simulink model "Problem_Simulation"  (R2023b)
settings: Solver=VariableStepAuto  StartTime=0.0  StopTime=1  RelTol=1e-3
libraries: spsDiodeLib x4, spsSeriesRLCBranchLib x2, spsTHDLib x2, spsVoltageMeasurementLib x2, spsACVoltageSourceLib x1, spsCurrentMeasurementLib x1, spsMeanLib x1, spsPowerLib x1, sps_lib x1
settings Model: Creator=HP  LastModifiedBy=HP

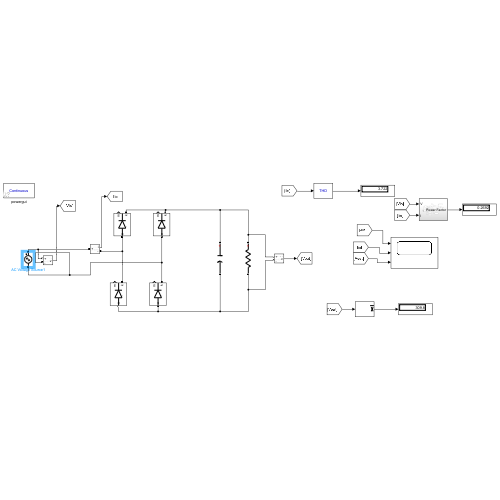
[thumbnail: Simulink's stored preview of the top-level diagram]
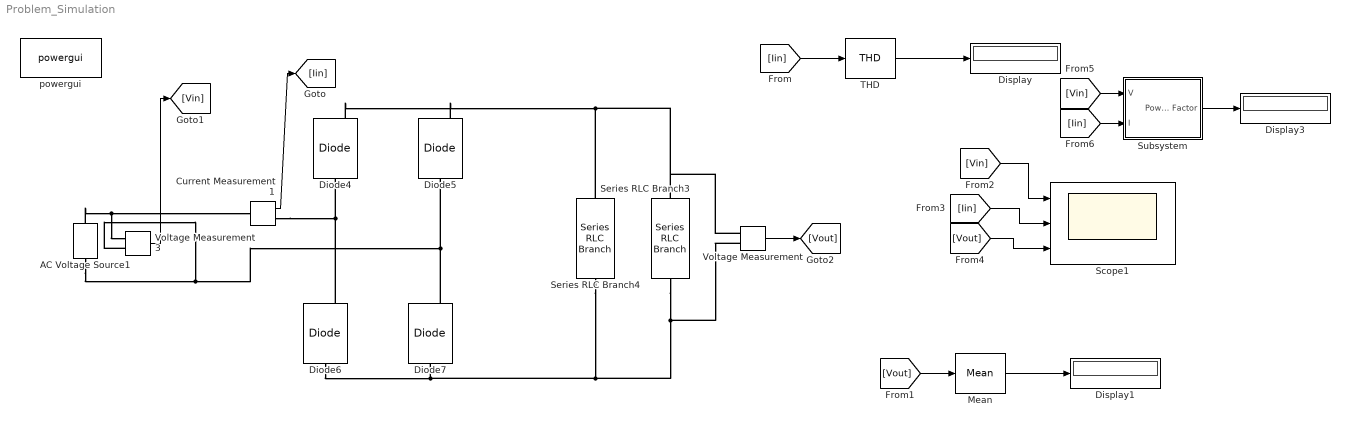
== system Problem_Simulation ==
  AC Voltage Source1 : spsACVoltageSourceLib/AC Voltage Source  Amplitude=220*sqrt(2)  Phase=0  Frequency=50  SampleTime=0  Measurements=None  BusType=swing  Pref=10e3  Qref=0  Qmin=-inf  Qmax=+inf
  Current Measurement1 : spsCurrentMeasurementLib/Current Measurement  PhasorSimulation=off  OutputType=Complex  PSBequivalent=0
  Diode{4..7} (4 alike) : spsDiodeLib/Diode  Ron=0.001  Lon=0  Vf=0.8  IC=0  UseSnubber=0  Rs=500  Cs=250e-9  Measurements=on
  Display : Display
  Display1 : Display
  Display3 : Display
  Mean : spsMeanLib/Mean  Freq=60  Vinit=0  Ts=0
  Scope1 : Scope  NumInputPorts=3
  Series RLC Branch3 : spsSeriesRLCBranchLib/Series RLC Branch  LConnTagsString=__new0  RConnTagsString=__new0  BranchType=R  Resistance=1000  Inductance=1e-3  SetiL0=off  InitialCurrent=0  Capacitance=1e-6  Setx0=off  InitialVoltage=0  Measurements=None
  Series RLC Branch4 : spsSeriesRLCBranchLib/Series RLC Branch  LConnTagsString=__new0  RConnTagsString=__new0  BranchType=C  Resistance=1  Inductance=1e-3  SetiL0=off  InitialCurrent=0  Capacitance=1000e-6  Setx0=off  InitialVoltage=0  Measurements=None
  Subsystem : Subsystem
  THD : spsTHDLib/THD  Freq=50  Ts=0
  Voltage Measurement : spsVoltageMeasurementLib/Voltage Measurement  PhasorSimulation=off  OutputType=Complex  PSBequivalent=0
  Voltage Measurement3 : spsVoltageMeasurementLib/Voltage Measurement  PhasorSimulation=off  OutputType=Complex  PSBequivalent=0
  powergui : sps_lib/powergui  Priority=1  SimulationMode=Continuous  SampleTime=50e-6  frequency=60  Iterations=50  frequencyindice=50  Pbase=100e6  ErrMax=1e-4  UnitsV=kV  UnitsW=MW  buscounter=0  FunctionMessages=off  echomessages=off  EnableUseOfTLC=off  CurrentSourceSwitches=off  DisableSnubberDevices=on  DisableRonSwitches=off  DisableVfSwitches=on  DisplayEquations=on  AutomaticDiscreteSolvers=off  SolverType=Tustin/Backward Euler (TBE)  Interpol=off  ExternalGateDelay=off  methode=off  Ts=100  x0status=blocks  SPID=on  SwTol=0  HookPort=off  NonlinearTolerance=1e-4  nMaxIteration=100  ContinueOnMaxIteration=off  RestoreLinks=warning  ResistiveCurrentMeasurement=off  Frange=[0:2:500]  Ylog=off  Xlog=on  ShowGrid=off  save=off  variable=ZData  structure=0  ZoomFFT=off  StartTime=0.0  cycles=1  DisplayStyle=1  fundamental=60  FreqAxis=off  MaxFrequency=1000  frequencyindicesteady=1  RmsSteady=1  display=off
  wires:
  THD/1 -> Display/1
  Subsystem/1(Power Factor) -> Display3/1
  Mean/1 -> Display1/1
  Current Measurement1/1 -> [Iin]
  [Iin] -> THD/1
  Voltage Measurement3/1 -> [Vin]
  Voltage Measurement/1 -> [Vout]
  [Vout] -> Mean/1
  [Vin] -> Scope1/1
  [Iin] -> Scope1/2
  [Vout] -> Scope1/3
  [Vin] -> Subsystem/1(V)
  [Iin] -> Subsystem/2(I)
  connections:
  Current Measurement1/RConn1 -- Diode4/LConn1 -- Diode6/RConn1
  Diode5/RConn1 -- Diode4/RConn1 -- Voltage Measurement/LConn1 -- Series RLC Branch3/LConn1 -- Series RLC Branch4/LConn1
  Series RLC Branch3/RConn1 -- Voltage Measurement/LConn2 -- Series RLC Branch4/RConn1 -- Diode7/LConn1 -- Diode6/LConn1
  AC Voltage Source1/RConn1 -- Voltage Measurement3/LConn1 -- Current Measurement1/LConn1
  AC Voltage Source1/LConn1 -- Voltage Measurement3/LConn2 -- Diode5/LConn1 -- Diode7/RConn1

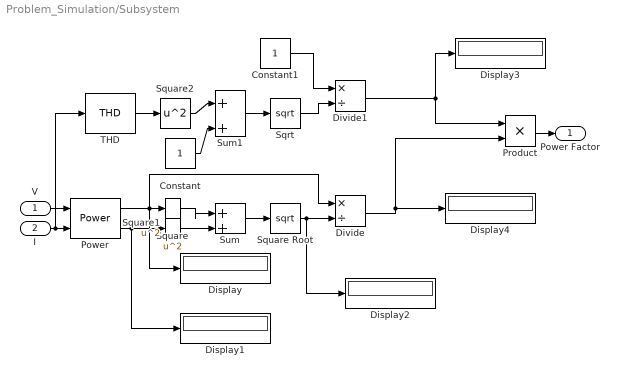
== system Problem_Simulation/Subsystem ==
  V : Inport
  I : Inport  Port=2
  Constant : Constant  SampleTime=-1
  Constant1 : Constant  SampleTime=-1
  Display{,1..4} (5 alike) : Display
  Divide : Product  Inputs=*/
  Divide1 : Product  Inputs=*/
  Power : spsPowerLib/Power  Freq=50  Vinit=[1, 0]  Iinit=[1, 0]  Ts=0
  Product : Product
  Sqrt : Sqrt
  Square : Math  Operator=square
  Square Root : Sqrt
  Square1 : Math  Operator=square
  Square2 : Math  Operator=square
  Sum : Sum  Inputs=|++
  Sum1 : Sum  Inputs=|++
  THD : spsTHDLib/THD  Freq=60  Ts=0
  Power Factor : Outport
  wires:
  Square/1 -> Sum/1
  Power/1 -> Divide/1, Display/1, Square/1
  Sum/1 -> Square Root/1
  Square Root/1 -> Divide/2, Display2/1
  Square1/1 -> Sum/2
  Power/2 -> Display1/1, Square1/1
  V/1 -> Power/1
  I/1 -> THD/1, Power/2
  Divide/1 -> Display4/1, Product/2
  Product/1 -> Power Factor/1
  THD/1 -> Square2/1
  Square2/1 -> Sum1/1
  Constant/1 -> Sum1/2
  Constant1/1 -> Divide1/1
  Sum1/1 -> Sqrt/1
  Sqrt/1 -> Divide1/2
  Divide1/1 -> Display3/1, Product/1
